simulink model "HDLHeaderRemoveRepetition"  (R2024a)
settings: Solver=VariableStepAuto  StartTime=0.0  StopTime=stopTime  RelTol=1e-3
undefined symbols (not defined in the file or in its folder): fs, headerBitsPerFec
libraries: dspsrcs4 x2, whdlutilities x2, hdlsllib x1
settings Model: Creator=cotti  LastModifiedBy=cotti

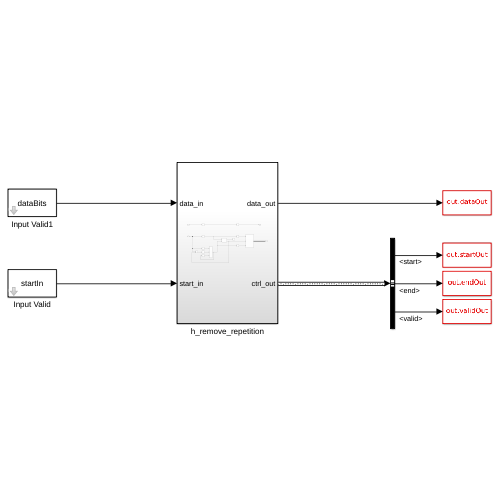
[thumbnail: Simulink's stored preview of the top-level diagram]
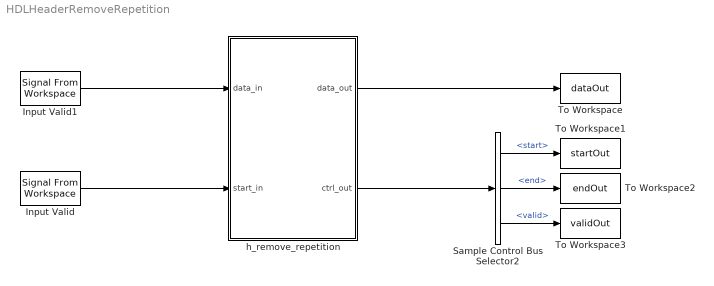
== system HDLHeaderRemoveRepetition ==
  Input Valid : dspsrcs4/Signal From Workspace  X=startIn  Ts=1/fs  nsamps=1  OutputAfterFinalValue=Setting to zero  ignoreOrWarnInputAndFrameLengths=off  OutputFrames=off
  Input Valid1 : dspsrcs4/Signal From Workspace  X=dataBits  Ts=1/fs  nsamps=1  OutputAfterFinalValue=Setting to zero  ignoreOrWarnInputAndFrameLengths=off  OutputFrames=off
  Sample Control Bus Selector2 : whdlutilities/Sample Control Bus Selector  OutputSignals=start,end,valid
  To Workspace : ToWorkspace  VariableName=dataOut  SampleTime=1/fs
      settings: Save2DSignal=2-D array (concatenate along first dimension)
  To Workspace1 : ToWorkspace  VariableName=startOut  SampleTime=1/fs
      settings: Save2DSignal=2-D array (concatenate along first dimension)
  To Workspace2 : ToWorkspace  VariableName=endOut  SampleTime=1/fs
      settings: Save2DSignal=2-D array (concatenate along first dimension)
  To Workspace3 : ToWorkspace  VariableName=validOut  SampleTime=1/fs
      settings: Save2DSignal=2-D array (concatenate along first dimension)
  h_remove_repetition : Subsystem
  wires:
  Input Valid/1 -> h_remove_repetition/2(start_in)
  Input Valid1/1 -> h_remove_repetition/1(data_in)
  h_remove_repetition/2(ctrl_out) -> Sample Control Bus Selector2/1
  Sample Control Bus Selector2/3 -> To Workspace3/1  "<valid>"
  h_remove_repetition/1(data_out) -> To Workspace/1
  Sample Control Bus Selector2/2 -> To Workspace2/1  "<end>"
  Sample Control Bus Selector2/1 -> To Workspace1/1  "<start>"

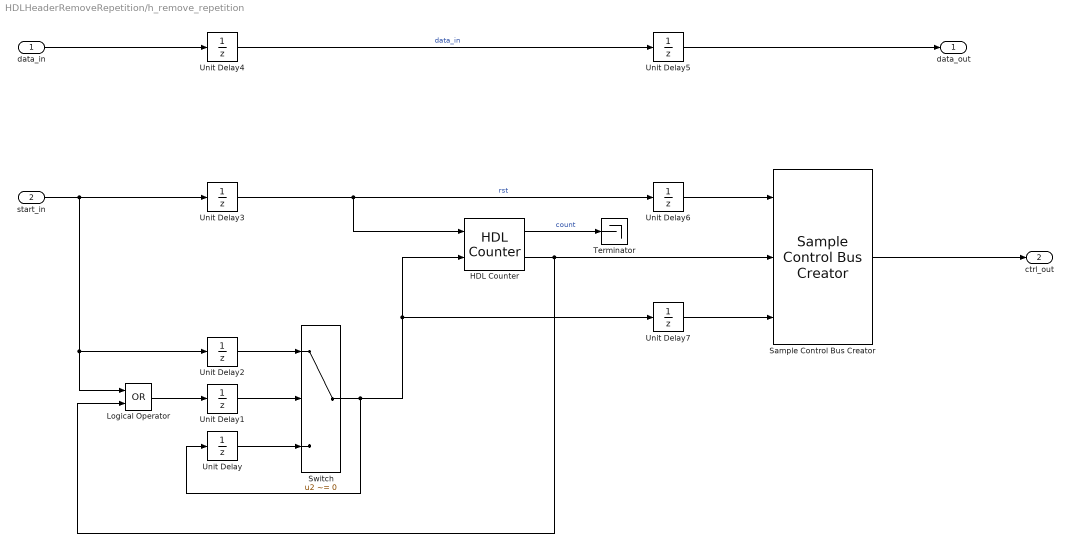
== system HDLHeaderRemoveRepetition/h_remove_repetition ==
  data_in : Inport
  start_in : Inport  Port=2
  HDL Counter : hdlsllib/Sources/HDL Counter  CountType=Count limited  CountInit=0  CountStep=1  CountMax=headerBitsPerFec-1  CountFromType=Initial value  CountFrom=0  CountResetPort=on  CountLoadPort=off  CountEnbPort=on  CountDirPort=off  CountHitOutputPort=on  CountDataType=Unsigned  CountWordLen=nextpow2(headerBitsPerFec)  CountFracLen=0  CountSampTime=1
  Logical Operator : Logic  Operator=OR  AllPortsSameDT=off  OutDataTypeStr=boolean
  Sample Control Bus Creator : whdlutilities/Sample Control Bus Creator
  Switch : Switch  Criteria=u2 ~= 0  SaturateOnIntegerOverflow=off  InputSameDT=off
  Terminator : Terminator
  Unit Delay{,1..7} (8 alike) : UnitDelay  SampleTime=-1  HasFrameUpgradeWarning=on
  data_out : Outport
  ctrl_out : Outport  Port=2
  wires:
  start_in/1 -> Unit Delay3/1, Logical Operator/1, Unit Delay2/1
  HDL Counter/2 -> Logical Operator/2, Sample Control Bus Creator/2
  data_in/1 -> Unit Delay4/1
  Sample Control Bus Creator/1 -> ctrl_out/1
  Unit Delay/1 -> Switch/3
  HDL Counter/1 -> Terminator/1  "count"
  Logical Operator/1 -> Unit Delay1/1
  Unit Delay1/1 -> Switch/2
  Unit Delay2/1 -> Switch/1
  Unit Delay4/1 -> Unit Delay5/1  "data_in"
  Unit Delay3/1 -> Unit Delay6/1, HDL Counter/1  "rst"
  Switch/1 -> Unit Delay7/1, HDL Counter/2, Unit Delay/1
  Unit Delay5/1 -> data_out/1
  Unit Delay6/1 -> Sample Control Bus Creator/1
  Unit Delay7/1 -> Sample Control Bus Creator/3
